simulink subsystem "ndi"  (R2024b)
settings: Solver=VariableStepAuto  StartTime=0.0  StopTime=10.0  RelTol=1e-3
undefined symbols (not defined in the file): k_alpha, wn_ndi_q, wn_ndi_r
settings Model: Creator=yagiz  LastModifiedBy=yagiz

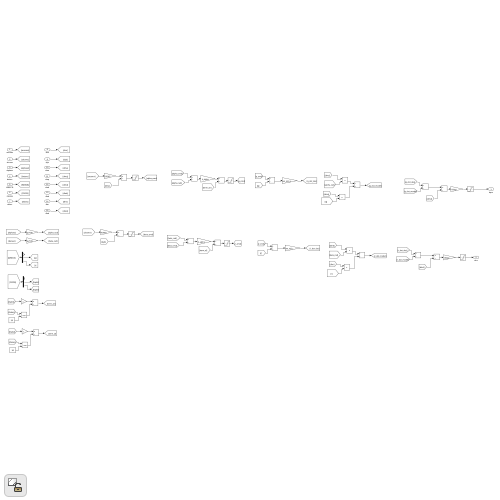
[thumbnail: Simulink's stored preview of the top-level diagram]
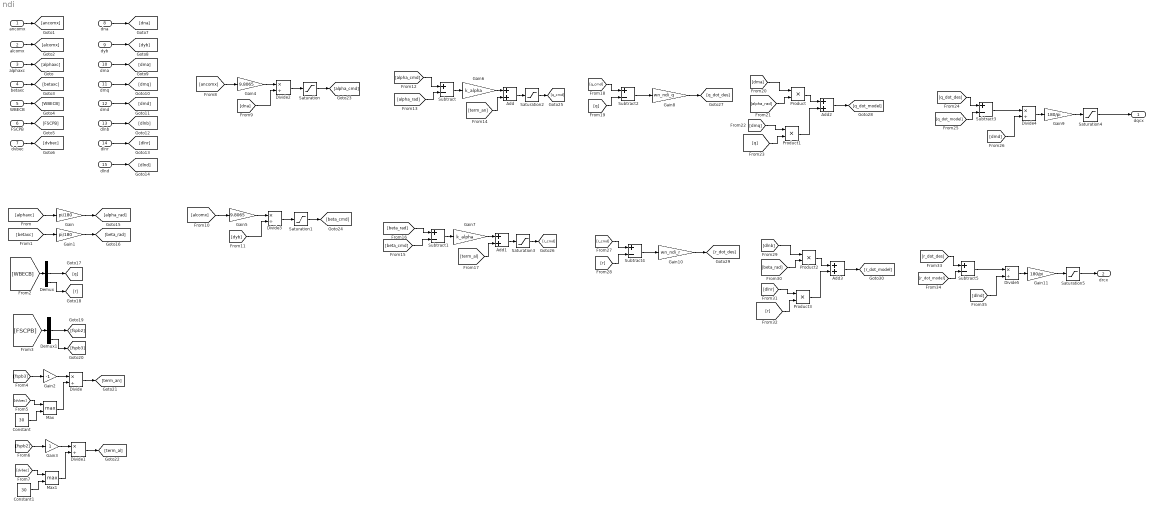
== system ndi ==
  ancomx : Inport
  alcomx : Inport  Port=2
  alphaxc : Inport  Port=3
  betaxc : Inport  Port=4
  WBECB : Inport  Port=5
  FSCPB : Inport  Port=6
  dvbec : Inport  Port=7
  dna : Inport  Port=8
  dyb : Inport  Port=9
  dma : Inport  Port=10
  dmq : Inport  Port=11
  dmd : Inport  Port=12
  dlnb : Inport  Port=13
  dlnr : Inport  Port=14
  dlnd : Inport  Port=15
  Add{,1..3} (4 alike) : Sum
  Constant : Constant  Value=30
  Constant1 : Constant  Value=30
  Demux : Demux  Outputs=3
  Demux1 : Demux  Outputs=3
  Divide{,1..5} (6 alike) : Product  Inputs=*/
  Gain : Gain  Gain=pi/180
  Gain1 : Gain  Gain=pi/180
  Gain10 : Gain  Gain=wn_ndi_r
  Gain11 : Gain  Gain=180/pi
  Gain2 : Gain  Gain=-1
  Gain3 : Gain
  Gain4 : Gain  Gain=9.8065
  Gain5 : Gain  Gain=9.8065
  Gain6 : Gain  Gain=k_alpha
  Gain7 : Gain  Gain=k_alpha
  Gain8 : Gain  Gain=wn_ndi_q
  Gain9 : Gain  Gain=180/pi
  Max : MinMax  Function=max  Inputs=2
  Max1 : MinMax  Function=max  Inputs=2
  Product{,1..3} (4 alike) : Product
  Saturation : Saturate  UpperLimit=0.803  LowerLimit=-0.803
  Saturation1 : Saturate  UpperLimit=0.803  LowerLimit=-0.803
  Saturation2 : Saturate  UpperLimit=0.524  LowerLimit=-0.524
  Saturation3 : Saturate  UpperLimit=0.524  LowerLimit=-0.524
  Saturation4 : Saturate  UpperLimit=28  LowerLimit=-280
  Saturation5 : Saturate  UpperLimit=28  LowerLimit=-280
  Subtract{,1..5} (6 alike) : Sum  Inputs=+-
  dqcx : Outport
  drcx : Outport  Port=2
  wires:
  alphaxc/1 -> [alphaxc]
  ancomx/1 -> [ancomx]
  alcomx/1 -> [alcomx]
  betaxc/1 -> [betaxc]
  WBECB/1 -> [WBECB]
  FSCPB/1 -> [FSCPB]
  dvbec/1 -> [dvbec]
  dna/1 -> [dna]
  dyb/1 -> [dyb]
  dma/1 -> [dma]
  dmq/1 -> [dmq]
  dmd/1 -> [dmd]
  dlnb/1 -> [dlnb]
  dlnr/1 -> [dlnr]
  dlnd/1 -> [dlnd]
  [alphaxc] -> Gain/1
  Gain/1 -> [alpha_rad]
  Gain1/1 -> [beta_rad]
  [betaxc] -> Gain1/1
  [WBECB] -> Demux/1
  Demux/2 -> [q]
  Demux/3 -> [r]
  Demux1/3 -> [fspb3]
  Demux1/2 -> [fspb2]
  [FSCPB] -> Demux1/1
  [fspb3] -> Gain2/1
  Gain2/1 -> Divide/1
  [dvbec] -> Max/1
  Constant/1 -> Max/2
  Max/1 -> Divide/2
  Divide/1 -> [term_an]
  Gain3/1 -> Divide1/1
  [dvbec] -> Max1/1
  [fspb2] -> Gain3/1
  Constant1/1 -> Max1/2
  Divide1/1 -> [term_al]
  Max1/1 -> Divide1/2
  [ancomx] -> Gain4/1
  Gain4/1 -> Divide2/1
  [dna] -> Divide2/2
  Divide2/1 -> Saturation/1
  Saturation/1 -> [alpha_cmd]
  [alcomx] -> Gain5/1
  Gain5/1 -> Divide3/1
  Divide3/1 -> Saturation1/1
  Saturation1/1 -> [beta_cmd]
  [dyb] -> Divide3/2
  [alpha_cmd] -> Subtract/1
  [alpha_rad] -> Subtract/2
  Subtract/1 -> Gain6/1
  Gain6/1 -> Add/1
  [term_an] -> Add/2
  Add/1 -> Saturation2/1
  Saturation2/1 -> [q_cmd]
  Add1/1 -> Saturation3/1
  Saturation3/1 -> [r_cmd]
  Subtract1/1 -> Gain7/1
  [term_al] -> Add1/2
  Gain7/1 -> Add1/1
  [q_cmd] -> Subtract2/1
  [q] -> Subtract2/2
  Subtract2/1 -> Gain8/1
  Gain8/1 -> [q_dot_des]
  [dma] -> Product/1
  [alpha_rad] -> Product/2
  Product/1 -> Add2/1
  [dmq] -> Product1/1
  [q] -> Product1/2
  Product1/1 -> Add2/2
  Add2/1 -> [q_dot_model]
  [q_dot_des] -> Subtract3/1
  [q_dot_model] -> Subtract3/2
  Subtract3/1 -> Divide4/1
  [dmd] -> Divide4/2
  Divide4/1 -> Gain9/1
  Gain9/1 -> Saturation4/1
  Saturation4/1 -> dqcx/1
  Subtract4/1 -> Gain10/1
  Gain10/1 -> [r_dot_des]
  [r_cmd] -> Subtract4/1
  [r] -> Subtract4/2
  [dlnb] -> Product2/1
  Add3/1 -> [r_dot_model]
  Product3/1 -> Add3/2
  Product2/1 -> Add3/1
  [dlnr] -> Product3/1
  [r] -> Product3/2
  [beta_rad] -> Product2/2
  [r_dot_des] -> Subtract5/1
  Gain11/1 -> Saturation5/1
  [dlnd] -> Divide5/2
  Subtract5/1 -> Divide5/1
  [r_dot_model] -> Subtract5/2
  Divide5/1 -> Gain11/1
  Saturation5/1 -> drcx/1
  [beta_rad] -> Subtract1/1
  [beta_cmd] -> Subtract1/2
